simulink model "LAB1_RMS_POWER"  (R2016b)
settings: Solver=VariableStepAuto  StartTime=0.0  StopTime=.00017  RelTol=1e-3
libraries: dspstat3 x1
settings Model: Creator=avile  LastModifiedBy=avile

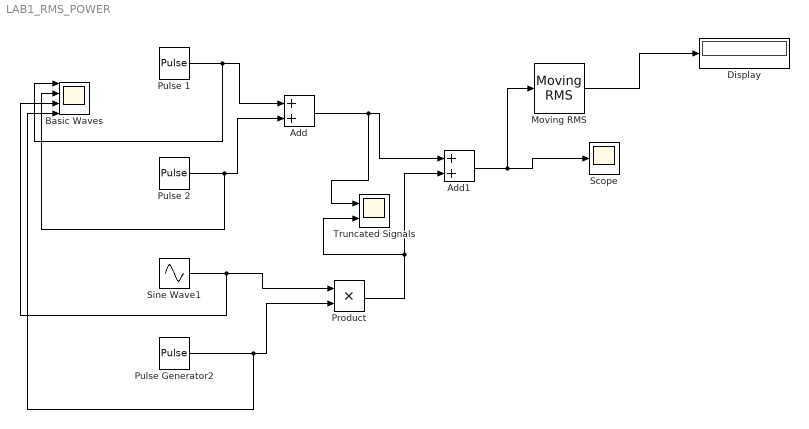
== system LAB1_RMS_POWER ==
  Add : Sum
  Add1 : Sum
  Basic Waves : Scope  NumInputPorts=4
  Display : Display
  Moving RMS : dspstat3/Moving RMS  Method=Sliding window  SpecifyWindowLength=on  WindowLength=4  ForgettingFactor=0.9  SimulateUsing=Code generation
  Product : Product
  "Pulse 1 " : DiscretePulseGenerator  PulseType=Time based  Amplitude=11  Period=.00017  PulseWidth=44  PhaseDelay=.0000408
  Pulse 2 : DiscretePulseGenerator  PulseType=Time based  Amplitude=-11  Period=.00017  PulseWidth=32  PhaseDelay=.0001156
  Pulse Generator2 : DiscretePulseGenerator  PulseType=Time based  Period=.00017  PulseWidth=24
  Scope : Scope
  Sine Wave1 : Sin  Amplitude=11  Frequency=6127*2*pi  SampleTime=0
  Truncated Signals : Scope  NumInputPorts=2
  wires:
  "Pulse 1 "/1 -> Basic Waves/1, Add/1
  Pulse 2/1 -> Basic Waves/2, Add/2
  Sine Wave1/1 -> Basic Waves/3, Product/1
  Pulse Generator2/1 -> Basic Waves/4, Product/2
  Add/1 -> Truncated Signals/1, Add1/1
  Moving RMS/1 -> Display/1
  Add1/1 -> Moving RMS/1, Scope/1
  Product/1 -> Truncated Signals/2, Add1/2
